simulink model "VTOLsimulink"  (R2017b)
settings: Solver=VariableStepAuto  StartTime=0.0  StopTime=10.0  RelTol=1e-3
values from neighbouring files (symbols this model uses):
  A = double(vpa(simplify(subs(As, states, states_op))))    [VTOLscript.m]    (also in space state.mat = [0 0 0 0 0 0 0 0 0 0 0 0 ... (196 elements, 14x14)])
  A_reduced_obsv = [A(1:10, 1:10), A(1:10, 13:14); A(13:14, 1:10), A(13:14, 13:14)]    [VTOLscript.m]
  B = double(vpa(simplify(subs(Bs, inputs, inputs_op))))    [VTOLscript.m]    (also in space state.mat = [0 0 0 1.29590488771 0 6.21792791514 2.57065584855 0 0 0 0 0)
  B_ro = [B(1:10, 1:end); B(13:14, 1:end)]    [VTOLscript.m]
  C = [1 zeros(1, 13) ... (first row only)    [VTOLscript.m]    (also in space state.mat = [1 0 0 0 0 0 0 0 0 0 0 1 ... (70 elements, 5x14)])
  C_ro = [C_ro(1:end, 1:10), C_ro(1:end, 13:14)]    [VTOLscript.m]
  D = [-10, zeros(1, 4); 0, -11, zeros(1, 3); zeros(1, 2), -12, zeros(1, 2); zeros(1, 3), -13, zeros(1, 1); zeros(1, 4), -14]    [VTOLscript.m]
  F1 = FF(1:12, 1:7)    [VTOLscript.m]
  F2 = FF(1:12, 8:end)    [VTOLscript.m]
  K = [G(1:end,1:10),zeros(5,2),G(1:end,11:end)]    [VTOLscript.m]
  Kro = [K(1:end,1:10) K(1:end,13:end)]    [VTOLscript.m]
  L = [eye(n - l), Ltil] * inv(Q)    [VTOLscript.m]
  pGcl = pinv(Gcl)    [VTOLscript.m]
  R = diag([10,10,10,1,1])    [VTOLscript.m]
  scale = -1    [VTOLscript.m]
  T = Atil_12 + Ltil * Atil_22 - D*Ltil    [VTOLscript.m]
libraries: vrlib x5
settings Model: Creator=Roozbeh  LastModifiedBy=kian
settings CodeAppCC: StateflowObjectComments=on

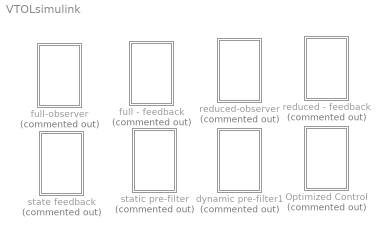
== system VTOLsimulink ==
  Optimized Control : Subsystem  Commented=on
  dynamic pre-filter1 : Subsystem  Commented=on
  "full - feedback " : Subsystem  Commented=on
  full-observer : Subsystem  Commented=on
  reduced - feedback : Subsystem  Commented=on
  reduced-observer : Subsystem  Commented=on
  state feedback : Subsystem  Commented=on
  static pre-filter : Subsystem  Commented=on

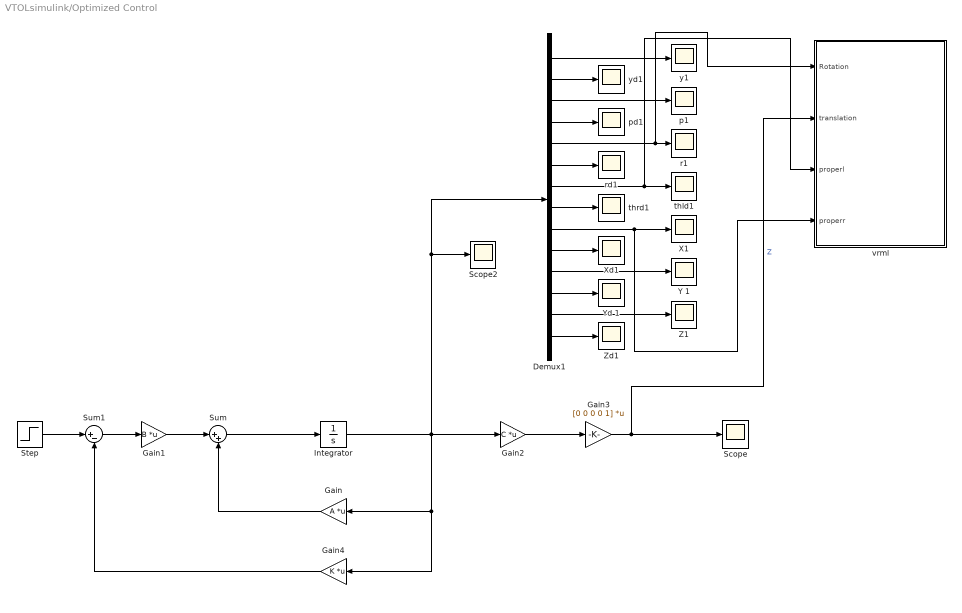
== system VTOLsimulink/Optimized Control ==
  Demux1 : Demux  Outputs=14
  Gain : Gain  Gain=A  Multiplication=Matrix(K*u)
  Gain1 : Gain  Gain=B  Multiplication=Matrix(K*u)
  Gain2 : Gain  Gain=C  Multiplication=Matrix(K*u)
  Gain3 : Gain  Gain=[0 0 0 0 1]  Multiplication=Matrix(K*u)
  Gain4 : Gain  Gain=K  Multiplication=Matrix(K*u)
  Integrator : Integrator  InitialCondition=zeros(14,1)
  Scope : Scope
  Scope2 : Scope
  Step : Step  Time=0  After=ones(5,1)  SampleTime=0
  Sum : Sum  Inputs=|++
  Sum1 : Sum  Inputs=|+-
  X1 : Scope
  Xd1 : Scope
  Y 1 : Scope
  Yd 1 : Scope
  Z1 : Scope
  Zd1 : Scope
  p1 : Scope
  pd1 : Scope
  r1 : Scope
  rd1 : Scope
  thld1 : Scope
  thrd1 : Scope
  vrml : Subsystem
  y1 : Scope
  yd1 : Scope
  wires:
  Sum1/1 -> Gain1/1
  Step/1 -> Sum1/1
  Gain1/1 -> Sum/1
  Gain4/1 -> Sum1/2
  Gain2/1 -> Gain3/1
  Sum/1 -> Integrator/1
  Gain/1 -> Sum/2
  Demux1/8 -> thrd1/1
  Demux1/1 -> y1/1
  Demux1/5 -> vrml/1("Rotation "), r1/1
  Demux1/14 -> Zd1/1
  Demux1/10 -> Xd1/1
  Demux1/12 -> Yd 1/1
  Demux1/13 -> Z1/1
  Gain3/1 -> vrml/2(translation), Scope/1  "Z"
  Demux1/9 -> vrml/4(properr), X1/1
  Demux1/2 -> yd1/1
  Demux1/7 -> vrml/3(properl), thld1/1
  Demux1/11 -> Y 1/1
  Demux1/6 -> rd1/1
  Demux1/3 -> p1/1
  Integrator/1 -> Demux1/1, Scope2/1, Gain2/1, Gain4/1, Gain/1
  Demux1/4 -> pd1/1

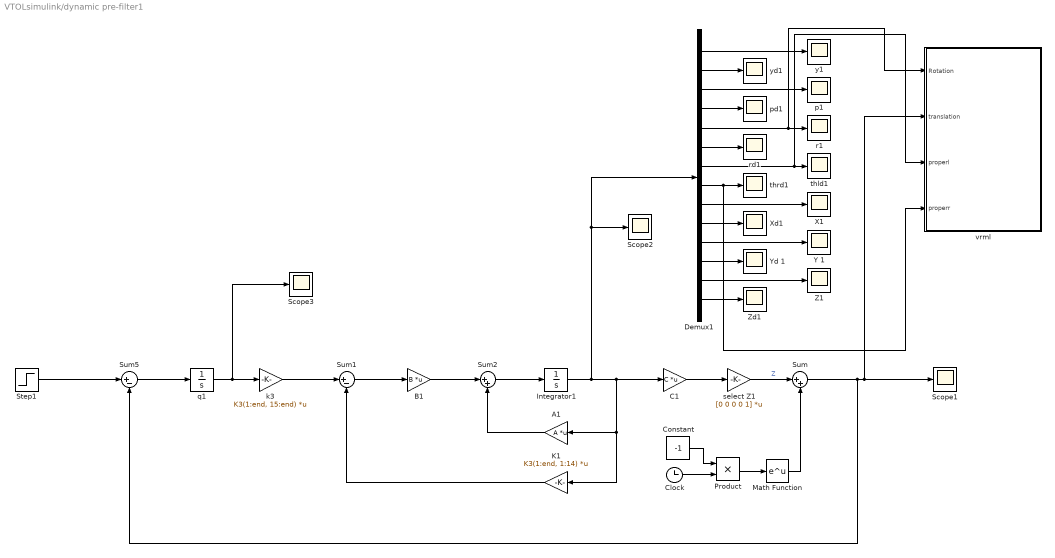
== system VTOLsimulink/dynamic pre-filter1 ==
  A1 : Gain  Gain=A  Multiplication=Matrix(K*u)
  B1 : Gain  Gain=B  Multiplication=Matrix(K*u)
  C1 : Gain  Gain=C  Multiplication=Matrix(K*u)
  Clock : Clock
  Constant : Constant  Value=-1
  Demux1 : Demux  Outputs=14
  Integrator1 : Integrator  InitialCondition=zeros(14,1)
  K1 : Gain  Gain=K3(1:end, 1:14)  Multiplication=Matrix(K*u)
  Math Function : Math  SaturateOnIntegerOverflow=on
  Product : Product
  Scope1 : Scope
  Scope2 : Scope
  Scope3 : Scope
  Step1 : Step  Time=0  After=5  SampleTime=0
  Sum : Sum  Inputs=|++
  Sum1 : Sum  Inputs=|+-
  Sum2 : Sum  Inputs=|++
  Sum5 : Sum  Inputs=|+-
  X1 : Scope
  Xd1 : Scope
  Y 1 : Scope
  Yd 1 : Scope
  Z1 : Scope
  Zd1 : Scope
  k3 : Gain  Gain=K3(1:end, 15:end)  Multiplication=Matrix(K*u)
  p1 : Scope
  pd1 : Scope
  q1 : Integrator
  r1 : Scope
  rd1 : Scope
  select Z1 : Gain  Gain=[0 0 0 0 1]  Multiplication=Matrix(K*u)
  thld1 : Scope
  thrd1 : Scope
  vrml : Subsystem
  y1 : Scope
  yd1 : Scope
  wires:
  K1/1 -> Sum1/2
  Sum1/1 -> B1/1
  Demux1/9 -> X1/1
  Demux1/5 -> vrml/1("Rotation "), r1/1
  Demux1/13 -> Z1/1
  Demux1/11 -> Y 1/1
  Demux1/6 -> rd1/1
  Demux1/7 -> vrml/3(properl), thld1/1
  Demux1/10 -> Xd1/1
  Demux1/8 -> vrml/4(properr), thrd1/1
  Demux1/12 -> Yd 1/1
  Demux1/14 -> Zd1/1
  Demux1/4 -> pd1/1
  Demux1/3 -> p1/1
  Demux1/2 -> yd1/1
  Demux1/1 -> y1/1
  A1/1 -> Sum2/2
  Sum2/1 -> Integrator1/1
  B1/1 -> Sum2/1
  Integrator1/1 -> Demux1/1, Scope2/1, C1/1, A1/1, K1/1
  Sum5/1 -> q1/1
  q1/1 -> Scope3/1, k3/1
  k3/1 -> Sum1/1
  Step1/1 -> Sum5/1
  C1/1 -> select Z1/1
  select Z1/1 -> Sum/1  "Z"
  Sum/1 -> Sum5/2, vrml/2(translation), Scope1/1
  Product/1 -> Math Function/1
  Clock/1 -> Product/2
  Constant/1 -> Product/1
  Math Function/1 -> Sum/2

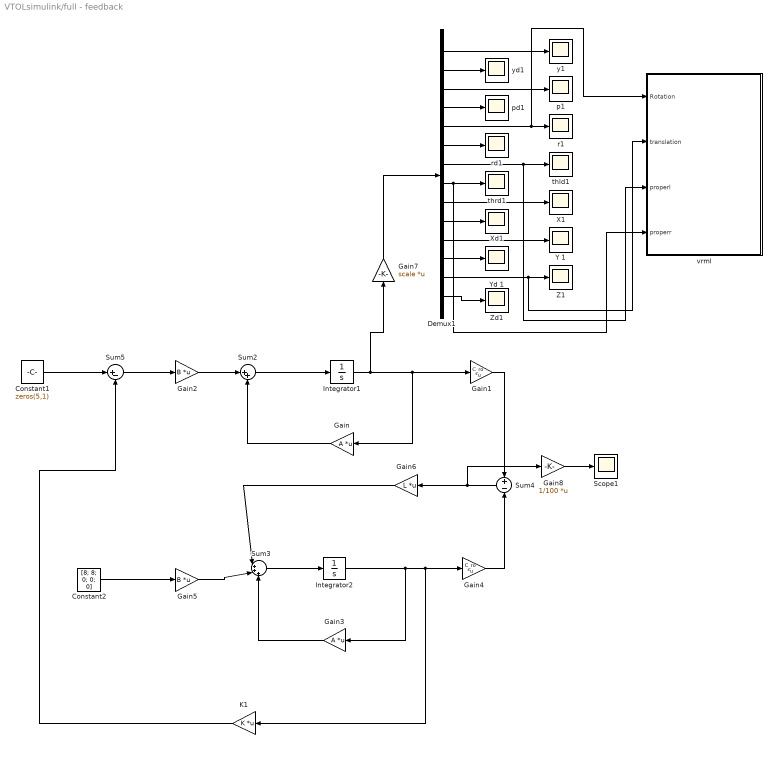
== system VTOLsimulink/full - feedback  ==
  Constant1 : Constant  Value=zeros(5,1)
  Constant2 : Constant  Value=[8; 8; 0; 0; 0]
  Demux1 : Demux  Outputs=14
  Gain : Gain  Gain=A  Multiplication=Matrix(K*u)
  Gain1 : Gain  Gain=C_ro  Multiplication=Matrix(K*u)
  Gain2 : Gain  Gain=B  Multiplication=Matrix(K*u)
  Gain3 : Gain  Gain=A  Multiplication=Matrix(K*u)
  Gain4 : Gain  Gain=C_ro  Multiplication=Matrix(K*u)
  Gain5 : Gain  Gain=B  Multiplication=Matrix(K*u)
  Gain6 : Gain  Gain=L  Multiplication=Matrix(K*u)
  Gain7 : Gain  Gain=scale  Multiplication=Matrix(K*u)
  Gain8 : Gain  Gain=1/100  Multiplication=Matrix(K*u)
  Integrator1 : Integrator  InitialCondition=[ones(1,10), 0, 0, 1, 1]
  Integrator2 : Integrator  InitialCondition=[3 2 8 12 4 6 7 1 3 -9 0 0 5 7]
  K1 : Gain  Gain=K  Multiplication=Matrix(K*u)
  Scope1 : Scope
  Sum2 : Sum  Inputs=|++
  Sum3 : Sum  Inputs=|+++
  Sum4 : Sum  Inputs=+-
  Sum5 : Sum  Inputs=|+-
  X1 : Scope
  Xd1 : Scope
  Y 1 : Scope
  Yd 1 : Scope
  Z1 : Scope
  Zd1 : Scope
  p1 : Scope
  pd1 : Scope
  r1 : Scope
  rd1 : Scope
  thld1 : Scope
  thrd1 : Scope
  vrml : Subsystem
  y1 : Scope
  yd1 : Scope
  wires:
  Gain2/1 -> Sum2/1
  Gain/1 -> Sum2/2
  Sum2/1 -> Integrator1/1
  Gain5/1 -> Sum3/2
  Integrator2/1 -> Gain3/1, K1/1, Gain4/1
  Sum3/1 -> Integrator2/1
  Gain1/1 -> Sum4/1
  Gain4/1 -> Sum4/2
  Sum4/1 -> Gain8/1, Gain6/1
  Gain6/1 -> Sum3/1
  Constant2/1 -> Gain5/1
  Gain3/1 -> Sum3/3
  Constant1/1 -> Sum5/1
  Sum5/1 -> Gain2/1
  K1/1 -> Sum5/2
  Demux1/5 -> vrml/1("Rotation "), r1/1
  Demux1/1 -> y1/1
  Demux1/9 -> X1/1
  Demux1/10 -> Xd1/1
  Demux1/7 -> vrml/3(properl), thld1/1
  Demux1/11 -> Y 1/1
  Demux1/3 -> p1/1
  Demux1/12 -> Yd 1/1
  Demux1/8 -> vrml/4(properr), thrd1/1
  Demux1/13 -> vrml/2(translation), Z1/1
  Demux1/14 -> Zd1/1
  Demux1/2 -> yd1/1
  Demux1/6 -> rd1/1
  Demux1/4 -> pd1/1
  Integrator1/1 -> Gain7/1, Gain1/1, Gain/1
  Gain7/1 -> Demux1/1
  Gain8/1 -> Scope1/1

== system VTOLsimulink/full-observer ==
  Constant : Constant  Value=[8; 8; 0; 0; 0]
  Constant1 : Constant  Value=[8; 8; 0; 0; 0]
  Gain : Gain  Gain=A  Multiplication=Matrix(K*u)
  Gain1 : Gain  Gain=C_ro  Multiplication=Matrix(K*u)
  Gain2 : Gain  Gain=B  Multiplication=Matrix(K*u)
  Gain3 : Gain  Gain=A  Multiplication=Matrix(K*u)
  Gain4 : Gain  Gain=C_ro  Multiplication=Matrix(K*u)
  Gain5 : Gain  Gain=B  Multiplication=Matrix(K*u)
  Gain6 : Gain  Gain=L  Multiplication=Matrix(K*u)
  Integrator : Integrator  InitialCondition=[ones(1,10), 0, 0, 1, 1]
  Integrator1 : Integrator  InitialCondition=[3 2 8 12 4 6 7 1 3 -9 0 0 5 7]
  Scope : Scope
  Sum : Sum  Inputs=|++
  Sum1 : Sum  Inputs=|+++
  Sum2 : Sum  Inputs=+-
  wires:
  Gain2/1 -> Sum/1
  Gain/1 -> Sum/2
  Sum/1 -> Integrator/1
  Gain5/1 -> Sum1/2
  Integrator1/1 -> Gain3/1, Gain4/1
  Sum1/1 -> Integrator1/1
  Gain1/1 -> Sum2/1
  Gain4/1 -> Sum2/2
  Sum2/1 -> Scope/1, Gain6/1
  Gain6/1 -> Sum1/1
  Constant/1 -> Gain2/1
  Constant1/1 -> Gain5/1
  Integrator/1 -> Gain1/1, Gain/1
  Gain3/1 -> Sum1/3

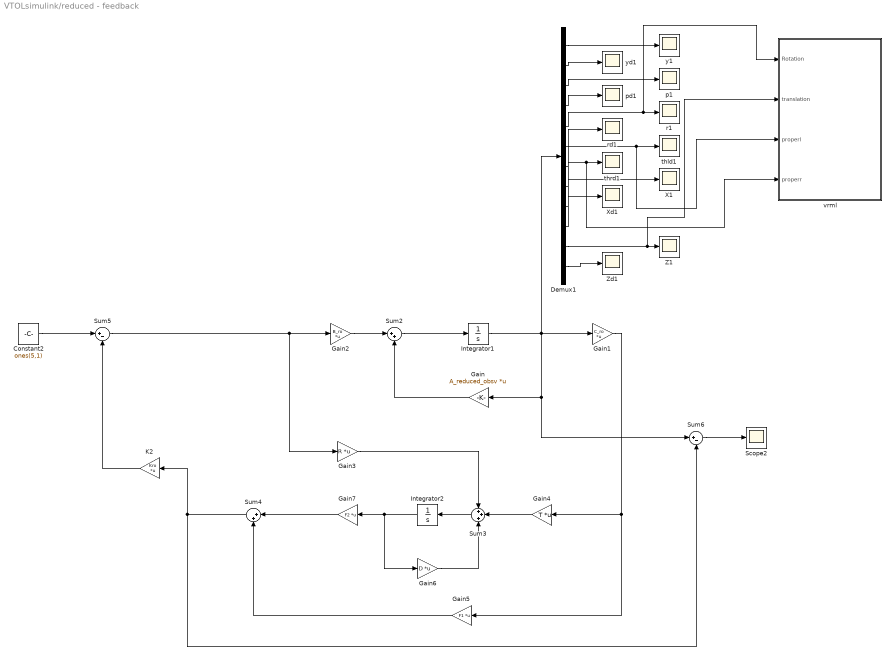
== system VTOLsimulink/reduced - feedback ==
  Constant2 : Constant  Value=ones(5,1)
  Demux1 : Demux  Outputs=12
  Gain : Gain  Gain=A_reduced_obsv  Multiplication=Matrix(K*u)
  Gain1 : Gain  Gain=C_ro  Multiplication=Matrix(K*u)
  Gain2 : Gain  Gain=B_ro  Multiplication=Matrix(K*u)
  Gain3 : Gain  Gain=R  Multiplication=Matrix(K*u)
  Gain4 : Gain  Gain=T  Multiplication=Matrix(K*u)
  Gain5 : Gain  Gain=F1  Multiplication=Matrix(K*u)
  Gain6 : Gain  Gain=D  Multiplication=Matrix(K*u)
  Gain7 : Gain  Gain=F2  Multiplication=Matrix(K*u)
  Integrator1 : Integrator  InitialCondition=[ones(1,10), 1, 1]
  Integrator2 : Integrator  InitialCondition=ones(5,1)
  K2 : Gain  Gain=Kro  Multiplication=Matrix(K*u)
  Scope2 : Scope
  Sum2 : Sum  Inputs=|++
  Sum3 : Sum  Inputs=+++
  Sum4 : Sum  Inputs=|++
  Sum5 : Sum  Inputs=|+-
  Sum6 : Sum  Inputs=|+-
  X1 : Scope
  Xd1 : Scope
  Z1 : Scope
  Zd1 : Scope
  p1 : Scope
  pd1 : Scope
  r1 : Scope
  rd1 : Scope
  thld1 : Scope
  thrd1 : Scope
  "vrml " : Subsystem
  y1 : Scope
  yd1 : Scope
  wires:
  Sum2/1 -> Integrator1/1
  Sum5/1 -> Gain3/1, Gain2/1
  Gain/1 -> Sum2/2
  Gain2/1 -> Sum2/1
  Gain4/1 -> Sum3/2
  Gain3/1 -> Sum3/1
  Gain5/1 -> Sum4/2
  Sum3/1 -> Integrator2/1
  Integrator2/1 -> Gain7/1, Gain6/1
  Gain6/1 -> Sum3/3
  Gain7/1 -> Sum4/1
  Sum4/1 -> K2/1, Sum6/2
  Gain1/1 -> Gain5/1, Gain4/1
  Sum6/1 -> Scope2/1
  Constant2/1 -> Sum5/1
  K2/1 -> Sum5/2
  Demux1/5 -> "vrml "/1("Rotation "), r1/1
  Demux1/1 -> y1/1
  Demux1/9 -> X1/1
  Demux1/10 -> Xd1/1
  Demux1/7 -> "vrml "/3(properl), thld1/1
  Demux1/3 -> p1/1
  Demux1/8 -> "vrml "/4(properr), thrd1/1
  Demux1/11 -> "vrml "/2(translation), Z1/1
  Demux1/12 -> Zd1/1
  Demux1/2 -> yd1/1
  Demux1/6 -> rd1/1
  Demux1/4 -> pd1/1
  Integrator1/1 -> Demux1/1, Sum6/1, Gain/1, Gain1/1

== system VTOLsimulink/reduced-observer ==
  Constant : Constant  Value=[8; 8; 0; 0; 0]
  Gain : Gain  Gain=A_reduced_obsv  Multiplication=Matrix(K*u)
  Gain1 : Gain  Gain=C_ro  Multiplication=Matrix(K*u)
  Gain2 : Gain  Gain=B_ro  Multiplication=Matrix(K*u)
  Gain3 : Gain  Gain=R  Multiplication=Matrix(K*u)
  Gain4 : Gain  Gain=T  Multiplication=Matrix(K*u)
  Gain5 : Gain  Gain=F1  Multiplication=Matrix(K*u)
  Gain6 : Gain  Gain=D  Multiplication=Matrix(K*u)
  Gain7 : Gain  Gain=F2  Multiplication=Matrix(K*u)
  Integrator : Integrator  InitialCondition=[ones(1,10), 1, 1]
  Integrator1 : Integrator  InitialCondition=ones(5,1)
  Scope : Scope
  Scope1 : Scope
  Sum : Sum  Inputs=|++
  Sum1 : Sum  Inputs=+++
  Sum2 : Sum  Inputs=|++
  Sum3 : Sum  Inputs=-+
  Sum4 : Sum  Inputs=|+-
  wires:
  Sum/1 -> Integrator/1
  Constant/1 -> Gain3/1, Gain2/1
  Gain/1 -> Sum/2
  Gain2/1 -> Sum/1
  Integrator/1 -> Sum4/1, Gain/1, Sum3/1, Gain1/1
  Gain4/1 -> Sum1/2
  Gain3/1 -> Sum1/1
  Gain5/1 -> Sum2/2
  Sum1/1 -> Integrator1/1
  Integrator1/1 -> Gain7/1, Gain6/1
  Gain6/1 -> Sum1/3
  Gain7/1 -> Sum2/1
  Sum2/1 -> Sum4/2, Sum3/2
  Sum3/1 -> Scope/1
  Gain1/1 -> Gain5/1, Gain4/1
  Sum4/1 -> Scope1/1

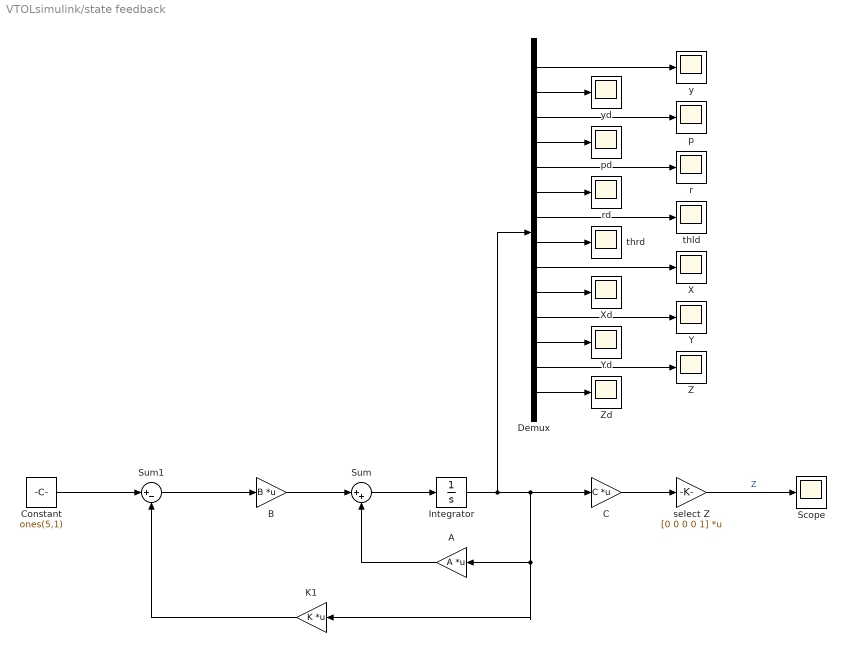
== system VTOLsimulink/state feedback ==
  A : Gain  Gain=A  Multiplication=Matrix(K*u)
  B : Gain  Gain=B  Multiplication=Matrix(K*u)
  C : Gain  Gain=C  Multiplication=Matrix(K*u)
  Constant : Constant  Value=ones(5,1)
  Demux : Demux  Outputs=14
  Integrator : Integrator  InitialCondition=zeros(14,1)
  K1 : Gain  Gain=K  Multiplication=Matrix(K*u)
  Scope : Scope
  Sum : Sum  Inputs=|++
  Sum1 : Sum  Inputs=|+-
  X : Scope
  Xd : Scope
  "Y " : Scope
  "Yd " : Scope
  Z : Scope
  Zd : Scope
  p : Scope
  pd : Scope
  r : Scope
  rd : Scope
  select Z : Gain  Gain=[0 0 0 0 1]  Multiplication=Matrix(K*u)
  thld : Scope
  thrd : Scope
  y : Scope
  yd : Scope
  wires:
  Integrator/1 -> Demux/1, C/1, K1/1, A/1
  A/1 -> Sum/2
  Constant/1 -> Sum1/1
  Demux/4 -> pd/1
  Sum1/1 -> B/1
  Sum/1 -> Integrator/1
  Demux/6 -> rd/1
  B/1 -> Sum/1
  select Z/1 -> Scope/1  "Z"
  C/1 -> select Z/1
  Demux/2 -> yd/1
  Demux/14 -> Zd/1
  Demux/13 -> Z/1
  Demux/8 -> thrd/1
  Demux/12 -> "Yd "/1
  Demux/3 -> p/1
  Demux/11 -> "Y "/1
  Demux/7 -> thld/1
  Demux/10 -> Xd/1
  Demux/9 -> X/1
  Demux/1 -> y/1
  Demux/5 -> r/1
  K1/1 -> Sum1/2

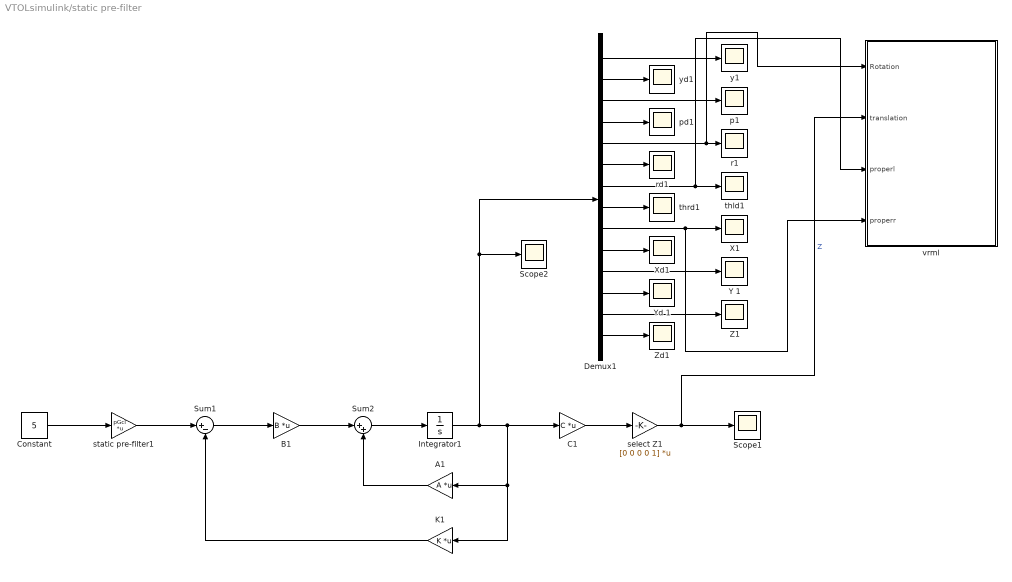
== system VTOLsimulink/static pre-filter ==
  A1 : Gain  Gain=A  Multiplication=Matrix(K*u)
  B1 : Gain  Gain=B  Multiplication=Matrix(K*u)
  C1 : Gain  Gain=C  Multiplication=Matrix(K*u)
  Constant : Constant  Value=5
  Demux1 : Demux  Outputs=14
  Integrator1 : Integrator  InitialCondition=zeros(14,1)
  K1 : Gain  Gain=K  Multiplication=Matrix(K*u)
  Scope1 : Scope
  Scope2 : Scope
  Sum1 : Sum  Inputs=|+-
  Sum2 : Sum  Inputs=|++
  X1 : Scope
  Xd1 : Scope
  Y 1 : Scope
  Yd 1 : Scope
  Z1 : Scope
  Zd1 : Scope
  p1 : Scope
  pd1 : Scope
  r1 : Scope
  rd1 : Scope
  select Z1 : Gain  Gain=[0 0 0 0 1]  Multiplication=Matrix(K*u)
  static pre-filter1 : Gain  Gain=pGcl  Multiplication=Matrix(K*u)
  thld1 : Scope
  thrd1 : Scope
  vrml : Subsystem
  y1 : Scope
  yd1 : Scope
  wires:
  Integrator1/1 -> K1/1, A1/1, C1/1, Scope2/1, Demux1/1
  B1/1 -> Sum2/1
  Sum2/1 -> Integrator1/1
  A1/1 -> Sum2/2
  Demux1/1 -> y1/1
  Demux1/2 -> yd1/1
  Demux1/3 -> p1/1
  C1/1 -> select Z1/1
  Demux1/4 -> pd1/1
  select Z1/1 -> vrml/2(translation), Scope1/1  "Z"
  Demux1/14 -> Zd1/1
  Demux1/12 -> Yd 1/1
  Demux1/10 -> Xd1/1
  Demux1/7 -> vrml/3(properl), thld1/1
  Demux1/6 -> rd1/1
  Demux1/11 -> Y 1/1
  Demux1/13 -> Z1/1
  Demux1/9 -> vrml/4(properr), X1/1
  Sum1/1 -> B1/1
  K1/1 -> Sum1/2
  static pre-filter1/1 -> Sum1/1
  Constant/1 -> static pre-filter1/1
  Demux1/5 -> vrml/1("Rotation "), r1/1
  Demux1/8 -> thrd1/1

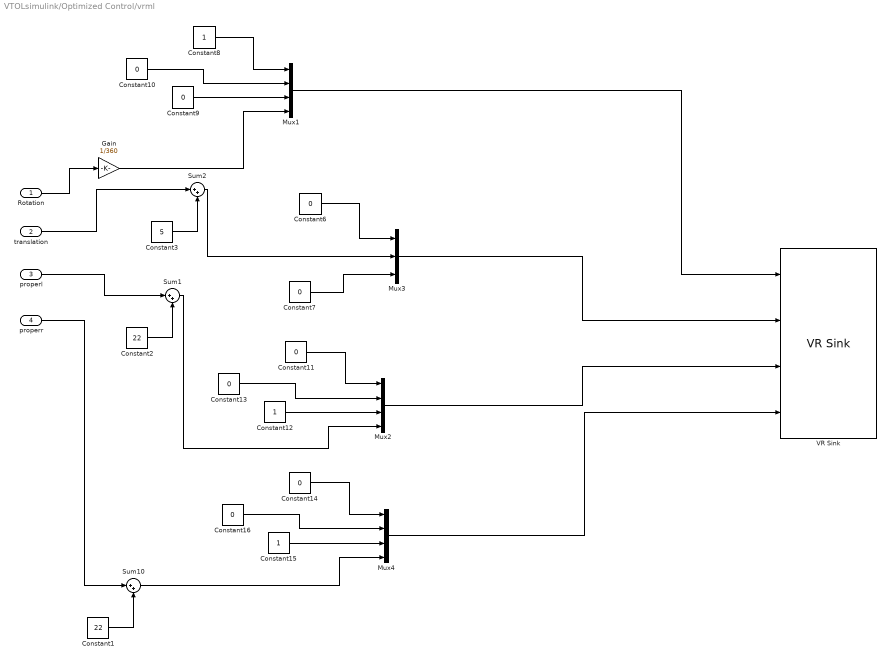
== system VTOLsimulink/Optimized Control/vrml ==
  "Rotation " : Inport
  translation : Inport  Port=2
  properl : Inport  Port=3
  properr : Inport  Port=4
  Constant1 : Constant  Value=22
  Constant{6..7,9..11,13..14,16} (8 alike) : Constant  Value=0
  Constant12 : Constant
  Constant15 : Constant
  Constant2 : Constant  Value=22
  Constant3 : Constant  Value=5
  Constant8 : Constant
  Gain : Gain  Gain=1/360
  Mux1 : Mux
  Mux2 : Mux
  Mux3 : Mux  Inputs=3
  Mux4 : Mux
  Sum1 : Sum  Inputs=|++
  Sum10 : Sum  Inputs=|++
  Sum2 : Sum  Inputs=|++
  VR Sink : vrlib/VR Sink  InstantiateOnLoad=on  SampleTime=0.1  ViewEnable=on  RemoteChange=off  RemoteView=off  FieldsWritten=V2Grp01.rotation.4.1.1.double#V2Grp01.translation.3.1.1.double#Left_Props.rotation.4.1.1.double#Right_Props.rotation.4.1.1.double  WorldFileName=vrml/osprey_all_1.WRL  AutoView=off  VideoDimensions=[]  AllowVariableSize=off
      settings: SourceProductBaseCode=VR
  wires:
  Constant11/1 -> Mux2/1
  Constant12/1 -> Mux2/3
  Constant13/1 -> Mux2/2
  Mux2/1 -> VR Sink/3
  Constant14/1 -> Mux4/1
  Constant15/1 -> Mux4/3
  Constant16/1 -> Mux4/2
  Mux4/1 -> VR Sink/4
  properr/1 -> Sum10/1
  Sum10/1 -> Mux4/4
  Constant1/1 -> Sum10/2
  Constant2/1 -> Sum1/2
  properl/1 -> Sum1/1
  Sum1/1 -> Mux2/4
  Constant6/1 -> Mux3/1
  Constant7/1 -> Mux3/3
  Mux3/1 -> VR Sink/2
  Constant3/1 -> Sum2/2
  Sum2/1 -> Mux3/2
  translation/1 -> Sum2/1
  Constant8/1 -> Mux1/1
  Constant9/1 -> Mux1/3
  Constant10/1 -> Mux1/2
  Gain/1 -> Mux1/4
  Mux1/1 -> VR Sink/1
  "Rotation "/1 -> Gain/1

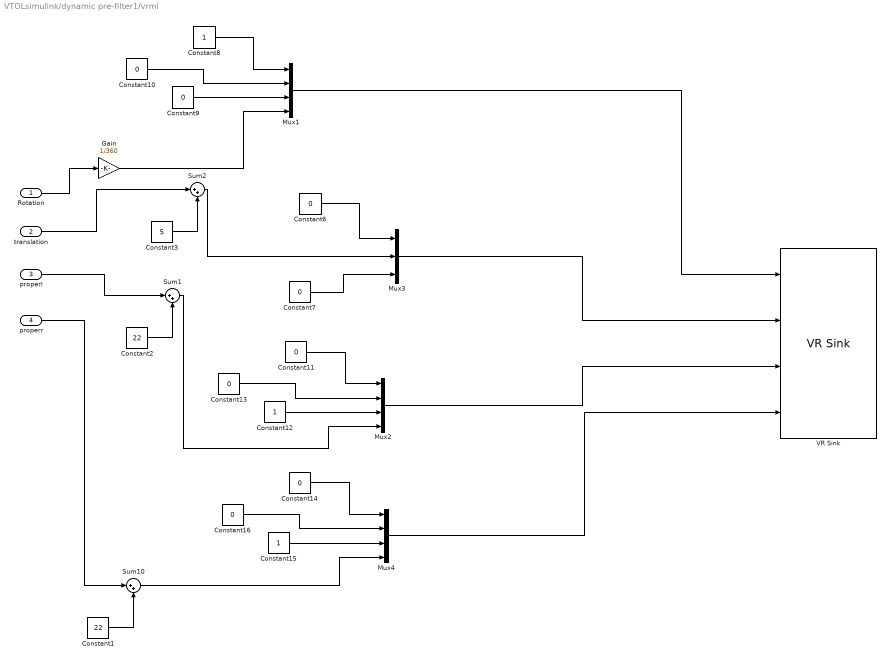
== system VTOLsimulink/dynamic pre-filter1/vrml ==
  "Rotation " : Inport
  translation : Inport  Port=2
  properl : Inport  Port=3
  properr : Inport  Port=4
  Constant1 : Constant  Value=22
  Constant{6..7,9..11,13..14,16} (8 alike) : Constant  Value=0
  Constant12 : Constant
  Constant15 : Constant
  Constant2 : Constant  Value=22
  Constant3 : Constant  Value=5
  Constant8 : Constant
  Gain : Gain  Gain=1/360
  Mux1 : Mux
  Mux2 : Mux
  Mux3 : Mux  Inputs=3
  Mux4 : Mux
  Sum1 : Sum  Inputs=|++
  Sum10 : Sum  Inputs=|++
  Sum2 : Sum  Inputs=|++
  VR Sink : vrlib/VR Sink  InstantiateOnLoad=on  SampleTime=0.1  ViewEnable=on  RemoteChange=off  RemoteView=off  FieldsWritten=V2Grp01.rotation.4.1.1.double#V2Grp01.translation.3.1.1.double#Left_Props.rotation.4.1.1.double#Right_Props.rotation.4.1.1.double  WorldFileName=vrml/osprey_all_1.WRL  AutoView=off  VideoDimensions=[]  AllowVariableSize=off
      settings: SourceProductBaseCode=VR
  wires:
  Constant11/1 -> Mux2/1
  Constant12/1 -> Mux2/3
  Constant13/1 -> Mux2/2
  Mux2/1 -> VR Sink/3
  Constant14/1 -> Mux4/1
  Constant15/1 -> Mux4/3
  Constant16/1 -> Mux4/2
  Mux4/1 -> VR Sink/4
  properr/1 -> Sum10/1
  Sum10/1 -> Mux4/4
  Constant1/1 -> Sum10/2
  Constant2/1 -> Sum1/2
  properl/1 -> Sum1/1
  Sum1/1 -> Mux2/4
  Constant6/1 -> Mux3/1
  Constant7/1 -> Mux3/3
  Mux3/1 -> VR Sink/2
  Constant3/1 -> Sum2/2
  Sum2/1 -> Mux3/2
  translation/1 -> Sum2/1
  Constant8/1 -> Mux1/1
  Constant9/1 -> Mux1/3
  Constant10/1 -> Mux1/2
  Gain/1 -> Mux1/4
  Mux1/1 -> VR Sink/1
  "Rotation "/1 -> Gain/1

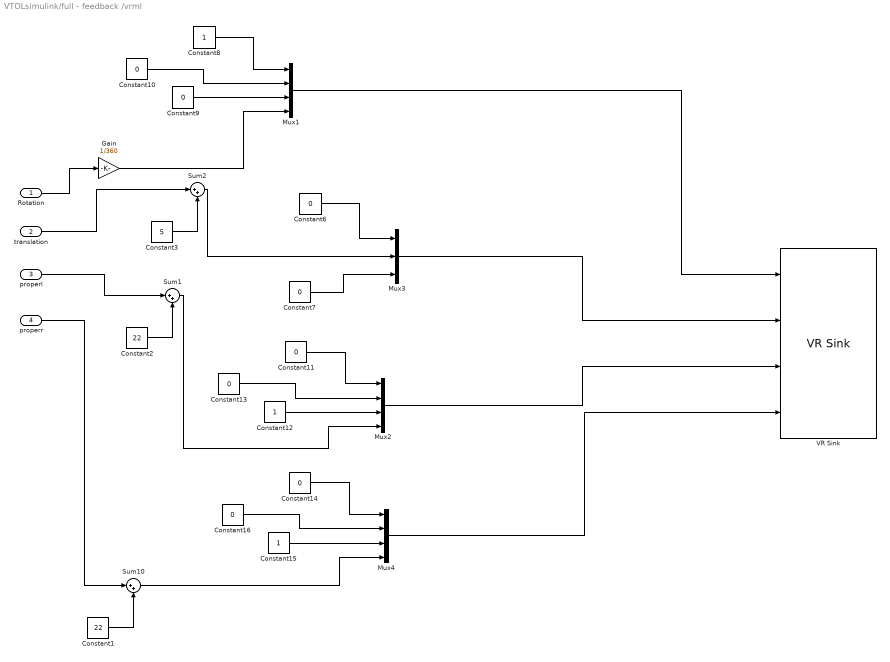
== system VTOLsimulink/full - feedback /vrml ==
  "Rotation " : Inport
  translation : Inport  Port=2
  properl : Inport  Port=3
  properr : Inport  Port=4
  Constant1 : Constant  Value=22
  Constant{6..7,9..11,13..14,16} (8 alike) : Constant  Value=0
  Constant12 : Constant
  Constant15 : Constant
  Constant2 : Constant  Value=22
  Constant3 : Constant  Value=5
  Constant8 : Constant
  Gain : Gain  Gain=1/360
  Mux1 : Mux
  Mux2 : Mux
  Mux3 : Mux  Inputs=3
  Mux4 : Mux
  Sum1 : Sum  Inputs=|++
  Sum10 : Sum  Inputs=|++
  Sum2 : Sum  Inputs=|++
  VR Sink : vrlib/VR Sink  InstantiateOnLoad=on  SampleTime=0.1  ViewEnable=on  RemoteChange=off  RemoteView=off  FieldsWritten=V2Grp01.rotation.4.1.1.double#V2Grp01.translation.3.1.1.double#Left_Props.rotation.4.1.1.double#Right_Props.rotation.4.1.1.double  WorldFileName=vrml/osprey_all_1.WRL  AutoView=off  VideoDimensions=[]  AllowVariableSize=off
      settings: SourceProductBaseCode=VR
  wires:
  Constant11/1 -> Mux2/1
  Constant12/1 -> Mux2/3
  Constant13/1 -> Mux2/2
  Mux2/1 -> VR Sink/3
  Constant14/1 -> Mux4/1
  Constant15/1 -> Mux4/3
  Constant16/1 -> Mux4/2
  Mux4/1 -> VR Sink/4
  properr/1 -> Sum10/1
  Sum10/1 -> Mux4/4
  Constant1/1 -> Sum10/2
  Constant2/1 -> Sum1/2
  properl/1 -> Sum1/1
  Sum1/1 -> Mux2/4
  Constant6/1 -> Mux3/1
  Constant7/1 -> Mux3/3
  Mux3/1 -> VR Sink/2
  Constant3/1 -> Sum2/2
  Sum2/1 -> Mux3/2
  translation/1 -> Sum2/1
  Constant8/1 -> Mux1/1
  Constant9/1 -> Mux1/3
  Constant10/1 -> Mux1/2
  Gain/1 -> Mux1/4
  Mux1/1 -> VR Sink/1
  "Rotation "/1 -> Gain/1

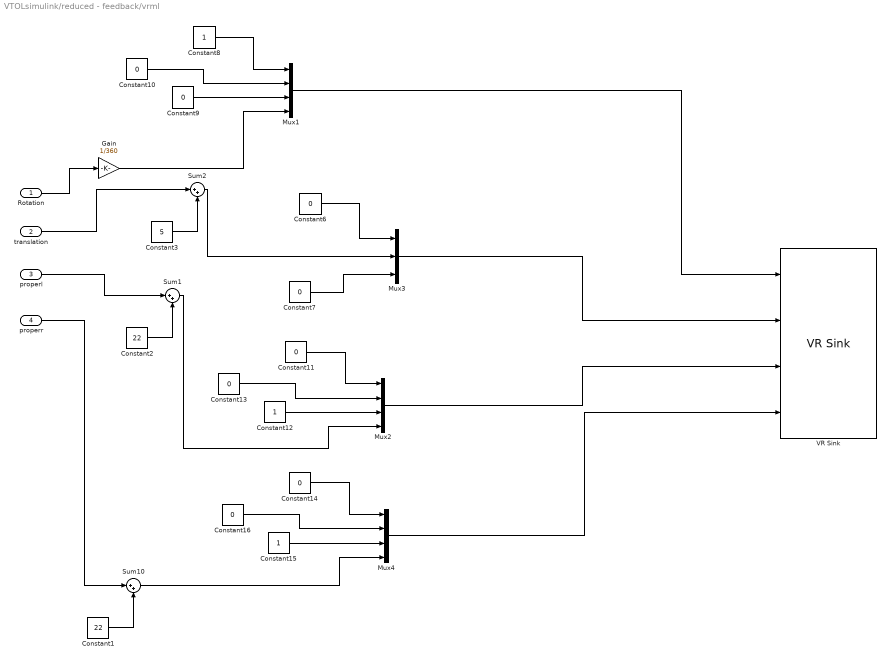
== system VTOLsimulink/reduced - feedback/vrml  ==
  "Rotation " : Inport
  translation : Inport  Port=2
  properl : Inport  Port=3
  properr : Inport  Port=4
  Constant1 : Constant  Value=22
  Constant{6..7,9..11,13..14,16} (8 alike) : Constant  Value=0
  Constant12 : Constant
  Constant15 : Constant
  Constant2 : Constant  Value=22
  Constant3 : Constant  Value=5
  Constant8 : Constant
  Gain : Gain  Gain=1/360
  Mux1 : Mux
  Mux2 : Mux
  Mux3 : Mux  Inputs=3
  Mux4 : Mux
  Sum1 : Sum  Inputs=|++
  Sum10 : Sum  Inputs=|++
  Sum2 : Sum  Inputs=|++
  VR Sink : vrlib/VR Sink  InstantiateOnLoad=on  SampleTime=0.1  ViewEnable=on  RemoteChange=off  RemoteView=off  FieldsWritten=V2Grp01.rotation.4.1.1.double#V2Grp01.translation.3.1.1.double#Left_Props.rotation.4.1.1.double#Right_Props.rotation.4.1.1.double  WorldFileName=vrml/osprey_all_1.WRL  AutoView=off  VideoDimensions=[]  AllowVariableSize=off
      settings: SourceProductBaseCode=VR
  wires:
  Constant11/1 -> Mux2/1
  Constant12/1 -> Mux2/3
  Constant13/1 -> Mux2/2
  Mux2/1 -> VR Sink/3
  Constant14/1 -> Mux4/1
  Constant15/1 -> Mux4/3
  Constant16/1 -> Mux4/2
  Mux4/1 -> VR Sink/4
  properr/1 -> Sum10/1
  Sum10/1 -> Mux4/4
  Constant1/1 -> Sum10/2
  Constant2/1 -> Sum1/2
  properl/1 -> Sum1/1
  Sum1/1 -> Mux2/4
  Constant6/1 -> Mux3/1
  Constant7/1 -> Mux3/3
  Mux3/1 -> VR Sink/2
  Constant3/1 -> Sum2/2
  Sum2/1 -> Mux3/2
  translation/1 -> Sum2/1
  Constant8/1 -> Mux1/1
  Constant9/1 -> Mux1/3
  Constant10/1 -> Mux1/2
  Gain/1 -> Mux1/4
  Mux1/1 -> VR Sink/1
  "Rotation "/1 -> Gain/1

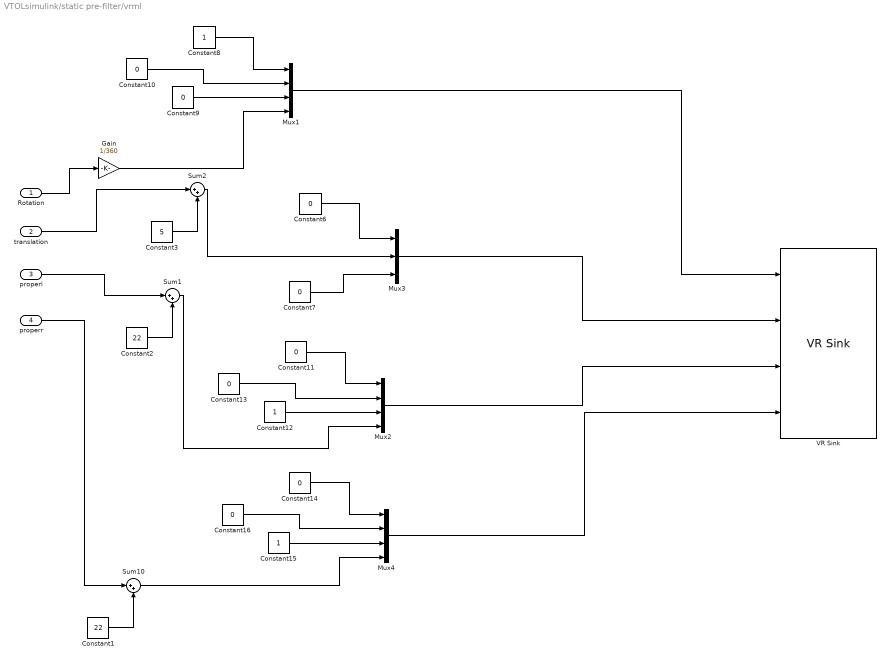
== system VTOLsimulink/static pre-filter/vrml ==
  "Rotation " : Inport
  translation : Inport  Port=2
  properl : Inport  Port=3
  properr : Inport  Port=4
  Constant1 : Constant  Value=22
  Constant{6..7,9..11,13..14,16} (8 alike) : Constant  Value=0
  Constant12 : Constant
  Constant15 : Constant
  Constant2 : Constant  Value=22
  Constant3 : Constant  Value=5
  Constant8 : Constant
  Gain : Gain  Gain=1/360
  Mux1 : Mux
  Mux2 : Mux
  Mux3 : Mux  Inputs=3
  Mux4 : Mux
  Sum1 : Sum  Inputs=|++
  Sum10 : Sum  Inputs=|++
  Sum2 : Sum  Inputs=|++
  VR Sink : vrlib/VR Sink  InstantiateOnLoad=on  SampleTime=0.1  ViewEnable=on  RemoteChange=off  RemoteView=off  FieldsWritten=V2Grp01.rotation.4.1.1.double#V2Grp01.translation.3.1.1.double#Left_Props.rotation.4.1.1.double#Right_Props.rotation.4.1.1.double  WorldFileName=vrml/osprey_all_1.WRL  AutoView=off  VideoDimensions=[]  AllowVariableSize=off
      settings: SourceProductBaseCode=VR
  wires:
  Constant11/1 -> Mux2/1
  Constant12/1 -> Mux2/3
  Constant13/1 -> Mux2/2
  Mux2/1 -> VR Sink/3
  Constant14/1 -> Mux4/1
  Constant15/1 -> Mux4/3
  Constant16/1 -> Mux4/2
  Mux4/1 -> VR Sink/4
  properr/1 -> Sum10/1
  Sum10/1 -> Mux4/4
  Constant1/1 -> Sum10/2
  Constant2/1 -> Sum1/2
  properl/1 -> Sum1/1
  Sum1/1 -> Mux2/4
  Constant6/1 -> Mux3/1
  Constant7/1 -> Mux3/3
  Mux3/1 -> VR Sink/2
  Constant3/1 -> Sum2/2
  Sum2/1 -> Mux3/2
  translation/1 -> Sum2/1
  Constant8/1 -> Mux1/1
  Constant9/1 -> Mux1/3
  Constant10/1 -> Mux1/2
  Gain/1 -> Mux1/4
  Mux1/1 -> VR Sink/1
  "Rotation "/1 -> Gain/1
